simulink model "fixed_wing_trajectory"  (R2023a)
settings: Solver=VariableStepAuto  StartTime=0.0  StopTime=75  RelTol=1e-3
undefined symbols (not defined in the file): Aircraft
libraries: simulink x2
settings Model: Creator=abhandari1  LastModifiedBy=abhandari1

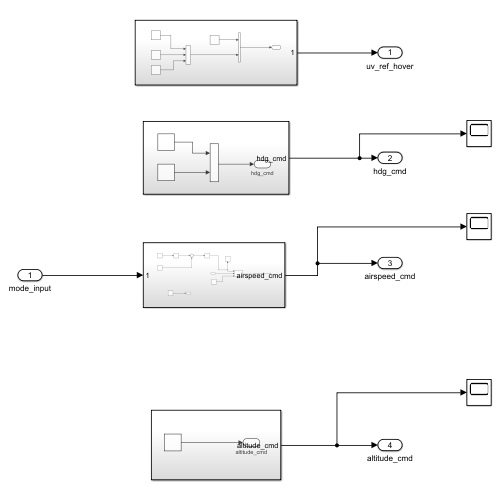
[thumbnail: Simulink's stored preview of the top-level diagram]
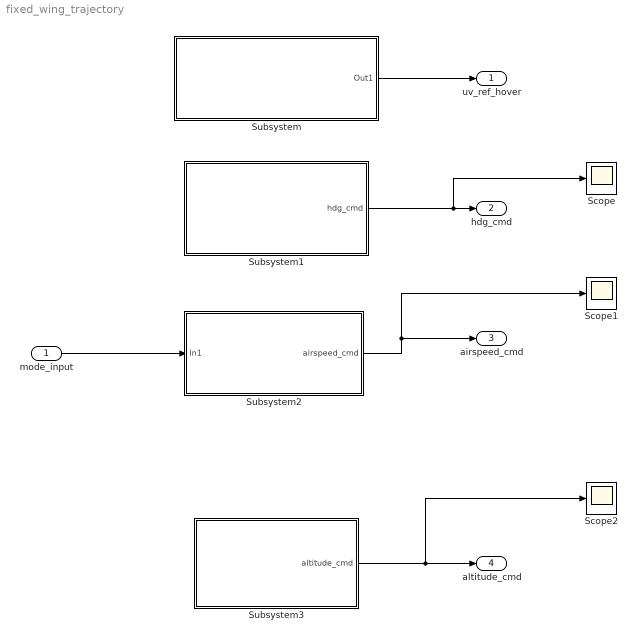
== system fixed_wing_trajectory ==
  mode_input : Inport
  Scope : Scope
  Scope1 : Scope
  Scope2 : Scope
  Subsystem : Subsystem
  Subsystem1 : Subsystem
  Subsystem2 : Subsystem
  Subsystem3 : Subsystem
  uv_ref_hover : Outport
  hdg_cmd : Outport  Port=2
  airspeed_cmd : Outport  Port=3
  altitude_cmd : Outport  Port=4
  wires:
  mode_input/1 -> Subsystem2/1(In1)
  Subsystem1/1(hdg_cmd) -> Scope/1, hdg_cmd/1
  Subsystem2/1(airspeed_cmd) -> Scope1/1, airspeed_cmd/1
  Subsystem3/1(altitude_cmd) -> Scope2/1, altitude_cmd/1
  Subsystem/1(Out1) -> uv_ref_hover/1

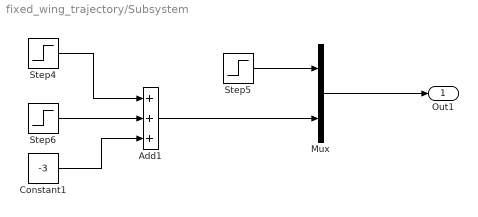
== system fixed_wing_trajectory/Subsystem ==
  Add1 : Sum  Inputs=+++
  Constant1 : Constant  Value=-3  OutDataTypeStr=single
  Mux : Mux  Inputs=2
  Step4 : Step  Time=4  After=3  OutDataTypeStr=single  SampleTime=0
  Step5 : Step  Time=27  After=0  OutDataTypeStr=single  SampleTime=0
  Step6 : Step  Time=7  Before=3  After=0  OutDataTypeStr=single  SampleTime=0
  Out1 : Outport
  wires:
  Step5/1 -> Mux/1
  Add1/1 -> Mux/2
  Step4/1 -> Add1/1
  Mux/1 -> Out1/1
  Constant1/1 -> Add1/3
  Step6/1 -> Add1/2

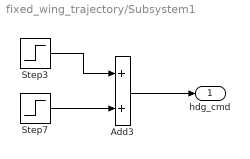
== system fixed_wing_trajectory/Subsystem1 ==
  Add3 : Sum
  Step3 : Step  Time=8  After=-1.2  OutDataTypeStr=single  SampleTime=0
  Step7 : Step  Time=25  After=1.8  OutDataTypeStr=single  SampleTime=0
  hdg_cmd : Outport
  wires:
  Step7/1 -> Add3/2
  Add3/1 -> hdg_cmd/1
  Step3/1 -> Add3/1

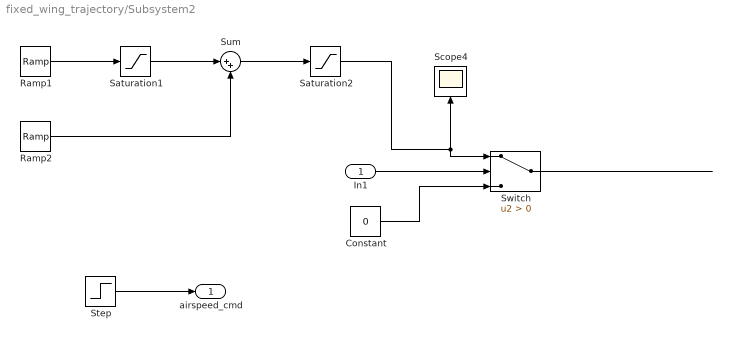
== system fixed_wing_trajectory/Subsystem2 ==
  In1 : Inport
  Constant : Constant  Value=0  OutDataTypeStr=single
  Ramp1 : simulink/Sources/Ramp  slope=Aircraft.Control.modes.hover2forward_airspeed_ramp  start=7  InitialOutput=0
  Ramp2 : simulink/Sources/Ramp  slope=Aircraft.Control.modes.forward2hover_airspeed_ramp  start=36  InitialOutput=0
  Saturation1 : Saturate  UpperLimit=22  LowerLimit=0  OutDataTypeStr=single
  Saturation2 : Saturate  UpperLimit=22  LowerLimit=0  OutDataTypeStr=single
  Scope4 : Scope
  Step : Step  Time=10  Before=20  After=25  OutDataTypeStr=single  SampleTime=0
  Sum : Sum  Inputs=|++
  Switch : Switch  Criteria=u2 > Threshold  SaturateOnIntegerOverflow=off  InputSameDT=off
  airspeed_cmd : Outport
  wires:
  Ramp1/1 -> Saturation1/1
  Constant/1 -> Switch/3
  Ramp2/1 -> Sum/2
  Saturation2/1 -> Switch/1, Scope4/1
  Sum/1 -> Saturation2/1
  Saturation1/1 -> Sum/1
  In1/1 -> Switch/2
  Switch/1 -> ?
  Step/1 -> airspeed_cmd/1

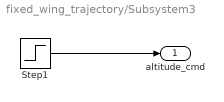
== system fixed_wing_trajectory/Subsystem3 ==
  Step1 : Step  Time=18  Before=100  After=90  OutDataTypeStr=single  SampleTime=0
  altitude_cmd : Outport
  wires:
  Step1/1 -> altitude_cmd/1
